simulink model "HLS_VMC_testing"  (R2025a)
settings: Solver=VariableStepAuto  StartTime=0.0  StopTime=0.0001  RelTol=1e-3
InitFcn:
  | fs = 500e6;
values from neighbouring files (symbols this model uses):
  N = length(X)    [outputPlots.m]
undefined symbols (not defined in the file or in its folder): A, es1, i, S, vsva2488, xcvr1602
libraries: hdlBasic x98, hlsBasic x64, aieUtilities x18, dspsrcs4 x15, dspxfrm3 x2, hdlDSPIP x2, hlsUtilities x1, vmcUtilities x1
(part 1 of 4)
settings Model: Creator=froregan  LastModifiedBy=froregan

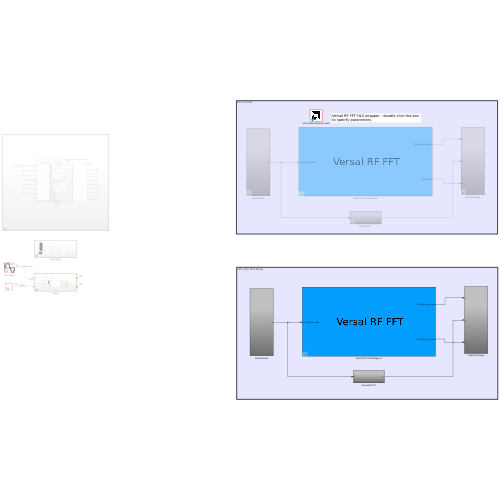
[thumbnail: Simulink's stored preview of the top-level diagram]
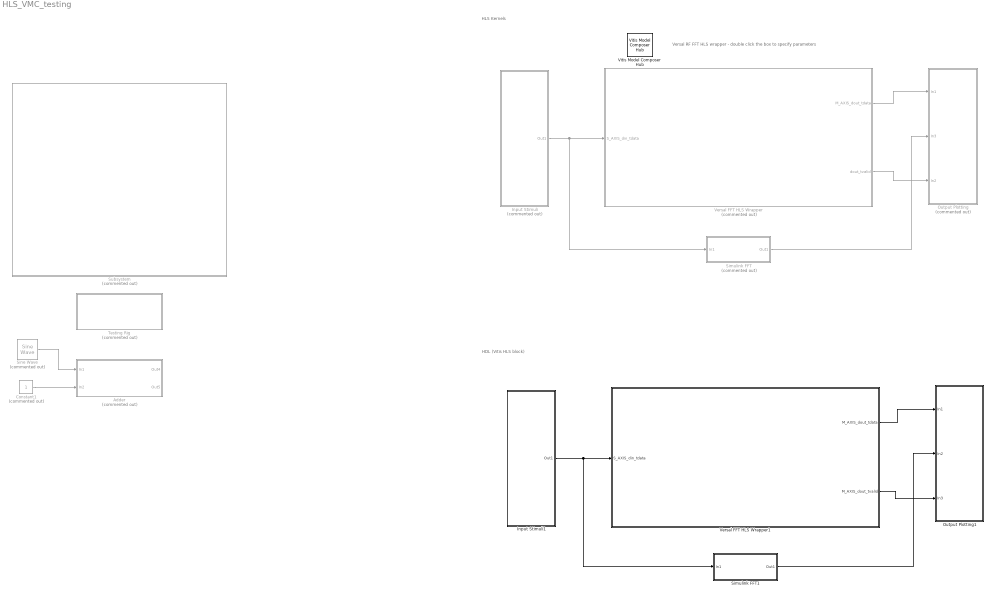
== system HLS_VMC_testing ==
  note: HDL (Vitis HLS block)
  note: HLS Kernels
  note: Versal RF FFT HLS wrapper - double click the box to specify parameters
  Adder : Subsystem  Commented=on
  Constant1 : Constant  Commented=on
  Input Stimuli : Subsystem  Commented=on
  Input Stimuli1 : Subsystem
  Output Plotting : Subsystem  Commented=on
  Output Plotting1 : Subsystem
  Simulink FFT : Subsystem  Commented=on
  Simulink FFT1 : Subsystem
  Sine Wave : dspsrcs4/Sine Wave  Commented=on  Amplitude=1  Frequency=100e6  Phase=0  SampleMode=Discrete  OutComplex=Real  CompMethod=Trigonometric fcn  TableSize=Speed  SampleTime=1/fs  SamplesPerFrame=1  ResetState=Restart at time zero  OutputFrames=off  dataType=double  wordLen=16  udDataType=sfix(16)  fracBitsMode=Best precision  numFracBits=15  OutDataTypeStr=double  LastOutDataTypeStr=double
  Subsystem : Subsystem  Commented=on
  Testing Rig : Subsystem  Commented=on
  Versal FFT HLS Wrapper : Subsystem  Commented=on  mask{tuser=1/1024, tuser_dir=IFFT, tuser_ps=10, FFT_SIZE=1024, sample_rate=SSR4, fft_max_point_size_temp=1024}
      mask prompts: tuser "TUSER Scaling"; tuser_dir "FFT Direction"; tuser_ps "TUSER Point Size"; FFT_SIZE "Period"; sample_rate "Super Sample Rate"; fft_max_point_size_temp "Maximum FFT Point Size"
      mask TypeOptions sample_rate: SSR2 | SSR4 | SSR8
      mask TypeOptions fft_max_point_size_temp: 16 | 32 | 64 | 128 | 256 | 512 | 1024 | 2048 | 4096
      mask DialogControl DescGroupVar Prompt: TUSER
      mask DialogControl Control4 Prompt: TUSER Scaling scales the output of the FFT
      mask DialogControl DescTextVar Prompt: TUSER Direction is either 1 for FFT or 0 for IFFT
      mask DialogControl Control3 Prompt: TUSER Point size is N where 2^N is the max FFT point size
      mask DialogControl ParameterGroupVar Prompt: TLAST
      mask DialogControl Control2 Prompt: Should be the same as the FFT size (in samples)
      mask DialogControl Container3 Prompt: Versal RF FFT
  Versal FFT HLS Wrapper1 : Subsystem  mask{tuser=1/1024, tuser_dir=FFT, tuser_ps=10, FFT_SIZE=1024, sample_rate=SSR4, fft_max_point_size_temp=1024}
      mask prompts: tuser "Scaling"; tuser_dir "FFT Direction"; tuser_ps "Point Size"; FFT_SIZE "Period"; sample_rate "Super Sample Rate"; fft_max_point_size_temp "Maximum FFT Point Size"
      mask TypeOptions sample_rate: SSR2 | SSR4 | SSR8
      mask TypeOptions fft_max_point_size_temp: 16 | 32 | 64 | 128 | 256 | 512 | 1024 | 2048 | 4096
      mask DialogControl DescGroupVar Prompt: TUSER
      mask DialogControl Control4 Prompt: TUSER Scaling scales the output of the FFT
      mask DialogControl DescTextVar Prompt: TUSER Direction is either 1 for FFT or 0 for IFFT
      mask DialogControl Control3 Prompt: TUSER Point size is N where 2^N is the max FFT point size
      mask DialogControl ParameterGroupVar Prompt: TLAST
      mask DialogControl Control2 Prompt: Should be the same as the FFT size (in samples)
      mask DialogControl Container3 Prompt: Versal RF FFT
  Vitis Model Composer Hub : vmcUtilities/Vitis Model Composer Hub  Tag=genX  CodeGeneration=off  SubsystemName=Versal FFT HLS Wrapper1  BlockHierPath=HLS_VMC_testing/Versal FFT HLS Wrapper1  CompilationType=HDLCompilation  SubsystemType=HDLNode  ExportTypeV2=IP Catalog  StartColumn=1  NumberOfColumns=1  TargetDirectory=./netlist  exportDesign=on  analyzeDesign=off  validateDesignOnHw=off  ExportType=AI Engines  IpVendor=xilinx.com  IpLibrary=hls  IpVersion=1.0  IpHWLanguage=Verilog  AieCompilerOptions={}  AieSimulatorOptions={}  CreateTestbench=off  TestbenchStackSize=10  RunRtlSim=off  RunCSim=off  RunAieSim=off  AieSimTimeout=50000  RunAieSimProfiling=off  LaunchVitisAnalyzer=off  PlotOutput=off  RunX86Sim=off  X86SimTimeout=10  GenHwImage=off  GenLibadfXo=on  GenHwValidationCode=off  PlatformType=Not Specified  HwSystemType=Baremetal  HwValidationTarget=hw  ProjDevice=xcvr1602-vsva2488-2HP-i-S-es1  ProjDevicePart=xcvr1602-vsva2488-2HP-i-S-es1  AIEType=AIE  SamplePeriod=-1  ClockFrequency=200  DataPathParallelism=1  xilinxfamily=versalairfes1  part=xcvr1602  speed=-2HP-i-S-es1  package=vsva2488  directory=./netlist/ip/Versal_FFT_HLS_Wrapper1/src  testbench=off  incr_netlist=off  synthesis_tool=Vivado  clock_wrapper=Clock Enables  dbl_ovrd=According to Block Masks  dcm_input_clock_period=10  sysclk_period=2  simulink_period=1/fs  eval_field=0  IPInfoJsonString="{\"DUTSubsystemName\":\"Versal FFT HLS Wrapper1\",\"HDLSubsystem\":{\"SubsystemName\":\"Versal_FFT_HLS_Wrapper1\",\"IPName\":\"Versal_FFT_HLS_Wrapper1\",\"IPLibrary\":\"VMC\",\"IPVendor\":\"User Company\",\"IPVersion\":\"1.0\",\"TargetDirectory\":\"./netlist\",\"SubsystemDir\":\"./netlist/ip/Versal_FFT_HLS_Wrapper1\",\"FreqHz\":\"500000000\"},\"SubsystemTag\":\"HDLNode\"}"  LogFileName=/proj/xirhdstaff1/froregan/icd7n/hegd_froregan_vmc_versalrf/DEV/hw/vmc_versalrf/HLS/netlist/model_composer.log  NThreads=4  IPConfigFile=/tmp/vmctmp-7794271613498057694/HLS_VMC_testing_ipconfig.json
  wires:
  Sine Wave/1 -> Adder/1(In1)
  Constant1/1 -> Adder/2(In2)
  Input Stimuli/1(Out1) -> Simulink FFT/1(In1), Versal FFT HLS Wrapper/1(S_AXIS_din_tdata)
  Versal FFT HLS Wrapper/1(M_AXIS_dout_tdata) -> Output Plotting/1(In1)
  Versal FFT HLS Wrapper/2(dout_tvalid) -> Output Plotting/3(In2)
  Simulink FFT/1(Out1) -> Output Plotting/2(In3)
  Simulink FFT1/1(Out1) -> Output Plotting1/2(In2)
  Input Stimuli1/1(Out1) -> Simulink FFT1/1(In1), Versal FFT HLS Wrapper1/1(S_AXIS_din_tdata)
  Versal FFT HLS Wrapper1/1(M_AXIS_dout_tdata) -> Output Plotting1/1(In1)
  Versal FFT HLS Wrapper1/2(M_AXIS_dout_tvalid) -> Output Plotting1/3(In3)

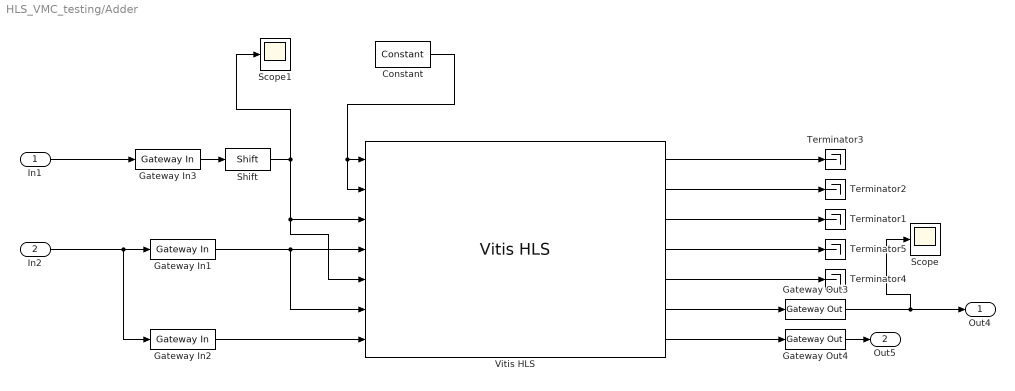
== system HLS_VMC_testing/Adder ==
  In1 : Inport
  In2 : Inport  Port=2
  Constant : hdlBasic/Constant  const=1.0  gui_display_data_type=Boolean  arith_type=Boolean  n_bits=16  bin_pt=14  preci_type=Single  exp_width=8  frac_width=24  explicit_period=off  period=1  XmcBlockStatus=1  maskContainerNames=tabcontainer1  block_type=constant  block_config=sysgen:Constant_config
  Gateway In1 : hdlBasic/Gateway In  gui_display_data_type=Boolean  arith_type=Boolean  n_bits=16  bin_pt=14  preci_type=Single  exp_width=8  frac_width=24  rows=1  columns=1  quantization="Round  (unbiased: +/- Inf)"  overflow=Saturate  period=1/fs  UseAsADC=off  ADCChannel='1'  interface=None  automatic_assignment=on  address_offset=hex2dec('00')  intf_name=''  intf_description=''  default_value=0  timing_constraint=None  locs_specified=off  LOCs={}  io_standard={}  inherit_from_input=off  hdl_port=on  XmcBlockStatus=1  maskContainerNames=group4  block_type=gatewayin  block_config=sysgen:gateway_in_config  block_width_w=590  block_height_w=620  block_width=640  block_height=850
  Gateway In2 : hdlBasic/Gateway In  gui_display_data_type=Boolean  arith_type=Boolean  n_bits=16  bin_pt=14  preci_type=Single  exp_width=8  frac_width=24  rows=1  columns=1  quantization="Round  (unbiased: +/- Inf)"  overflow=Saturate  period=1/fs  UseAsADC=off  ADCChannel='1'  interface=None  automatic_assignment=on  address_offset=hex2dec('00')  intf_name=''  intf_description=''  default_value=0  timing_constraint=None  locs_specified=off  LOCs={}  io_standard={}  inherit_from_input=off  hdl_port=on  XmcBlockStatus=1  maskContainerNames=group4  block_type=gatewayin  block_config=sysgen:gateway_in_config  block_width_w=590  block_height_w=620  block_width=640  block_height=850
  Gateway In3 : hdlBasic/Gateway In  gui_display_data_type=Fixed-point  arith_type=Signed (2's comp)  n_bits=32  bin_pt=31  preci_type=Single  exp_width=8  frac_width=24  rows=1  columns=1  quantization="Round  (unbiased: +/- Inf)"  overflow=Saturate  period=1/fs  UseAsADC=off  ADCChannel='1'  interface=None  automatic_assignment=on  address_offset=hex2dec('00')  intf_name=''  intf_description=''  default_value=0  timing_constraint=None  locs_specified=off  LOCs={}  io_standard={}  inherit_from_input=off  hdl_port=on  XmcBlockStatus=1  maskContainerNames=group4  block_type=gatewayin  block_config=sysgen:gateway_in_config  block_width_w=590  block_height_w=620  block_width=640  block_height=850
  Gateway Out3 : hdlBasic/Gateway Out  inherit_from_input=off  bool_to_boolean=off  hdl_port=on  rows=1  columns=1  UseAsDAC=off  DACChannel='1'  interface=None  automatic_assignment=on  address_offset=hex2dec('00')  intf_name=''  intf_description=''  timing_constraint=None  locs_specified=off  LOCs={}  io_standard={}  XmcBlockStatus=1  maskContainerNames=group4  block_type=gatewayout  block_config=sysgen:gateway_out_config  block_width_w=590  block_height_w=620  block_width=620  block_height=750
  Gateway Out4 : hdlBasic/Gateway Out  inherit_from_input=off  bool_to_boolean=off  hdl_port=on  rows=1  columns=1  UseAsDAC=off  DACChannel='1'  interface=None  automatic_assignment=on  address_offset=hex2dec('00')  intf_name=''  intf_description=''  timing_constraint=None  locs_specified=off  LOCs={}  io_standard={}  XmcBlockStatus=1  maskContainerNames=group4  block_type=gatewayout  block_config=sysgen:gateway_out_config  block_width_w=590  block_height_w=620  block_width=620  block_height=750
  Scope : Scope
      settings: ActiveDisplayYMinimum=-2.213061075E+9  ActiveDisplayYMaximum=2.213061075E+9  DataLoggingVariableName=ScopeData24
  Scope1 : Scope
      settings: ActiveDisplayYMinimum=-2.55297289625E+9  ActiveDisplayYMaximum=2.55297289625E+9  DataLoggingVariableName=ScopeData8
  Shift : hdlBasic/Shift  shift_dir=Left  shift_bits=31  en=off  latency=0  precision=User Defined  arith_type="Signed  (2's comp)"  n_bits=32  bin_pt=0  quantization=Truncate  overflow=Wrap  XmcBlockStatus=1  maskContainerNames=group2  block_type=shift  block_config=sysgen:Shift_config
  Terminator{1..5} (5 alike) : Terminator
  Vitis HLS : hdlBasic/Vitis HLS  anytable='/proj/xirhdstaff1/froregan/icd7n/hegd_froregan_vmc_versalrf/DEV/hw/vmc_versalrf/HLS/adder/adder/hls'  fast_sim=off  display_datatype=on  rate_propagation_method=Simulink system period  model_file_path=''  latency=1  block_type=vitis_hls
      settings: infoedit=This block allows including C,C++ and SystemC source files in System Generator for DSP designs.
  Out4 : Outport
  Out5 : Outport  Port=2
  wires:
  In1/1 -> Gateway In3/1
  In2/1 -> Gateway In2/1, Gateway In1/1
  Gateway In1/1 -> Vitis HLS/6, Vitis HLS/4
  Gateway In3/1 -> Shift/1
  Gateway In2/1 -> Vitis HLS/7
  Vitis HLS/6 -> Gateway Out3/1
  Gateway Out3/1 -> Scope/1, Out4/1
  Vitis HLS/7 -> Gateway Out4/1
  Gateway Out4/1 -> Out5/1
  Vitis HLS/2 -> Terminator2/1
  Vitis HLS/3 -> Terminator1/1
  Vitis HLS/1 -> Terminator3/1
  Vitis HLS/4 -> Terminator5/1
  Vitis HLS/5 -> Terminator4/1
  Shift/1 -> Vitis HLS/5, Vitis HLS/3, Scope1/1
  Constant/1 -> Vitis HLS/1, Vitis HLS/2

== system HLS_VMC_testing/Input Stimuli ==
  Chirp : dspsrcs4/Chirp  sweep=Quadratic  mode=Unidirectional  f0=100e3  f1=150e6  t1=1024/fs  Tsweep=1024/fs  phase=0  Ts=1/fs  spf=1  datatype=double  OutputFrames=off
  Chirp2 : dspsrcs4/Chirp  sweep=Quadratic  mode=Unidirectional  f0=100e3  f1=150e6  t1=1024/fs  Tsweep=1024/fs  phase=pi  Ts=1/fs  spf=1  datatype=double  OutputFrames=off
  Real-Imag to Complex : RealImagToComplex
  Sine Wave : dspsrcs4/Sine Wave  Commented=on  Amplitude=1  Frequency=100e3  Phase=0  SampleMode=Discrete  OutComplex=Complex  CompMethod=Trigonometric fcn  TableSize=Speed  SampleTime=1/fs  SamplesPerFrame=1  ResetState=Restart at time zero  OutputFrames=off  dataType=double  wordLen=16  udDataType=sfix(16)  fracBitsMode=Best precision  numFracBits=15  OutDataTypeStr=double  LastOutDataTypeStr=double
  Spectrum Analyzer : SpectrumAnalyzer  WindowPosition=[880.000000,470.000000,800.000000,500.000000,]  ScopeFrameLocation=window  WindowInvariantSamplesPerUpdate=on  Span=499999999.99999994  StartFrequency=-249999999.99999997  StopFrequency=249999999.99999997  YLimits=[-48.7308 24.4928]
  Out1 : Outport
  wires:
  Chirp2/1 -> Real-Imag to Complex/2
  Chirp/1 -> Real-Imag to Complex/1
  Real-Imag to Complex/1 -> Spectrum Analyzer/1, Out1/1

== system HLS_VMC_testing/Input Stimuli1 ==
  Chirp : dspsrcs4/Chirp  sweep=Quadratic  mode=Unidirectional  f0=100e3  f1=150e6  t1=1024/fs  Tsweep=1024/fs  phase=0  Ts=1/fs  spf=1  datatype=double  OutputFrames=off
  Chirp2 : dspsrcs4/Chirp  sweep=Quadratic  mode=Unidirectional  f0=100e3  f1=150e6  t1=1024/fs  Tsweep=1024/fs  phase=pi  Ts=1/fs  spf=1  datatype=double  OutputFrames=off
  Pre Processing : Subsystem
  Scope : Scope
      settings: ActiveDisplayYMinimum=-1.1949385808320478  ActiveDisplayYMaximum=1.2438820645368942  DataLoggingVariableName=ScopeData12
  Sine Wave : dspsrcs4/Sine Wave  Amplitude=1  Frequency=100e6  Phase=0  SampleMode=Discrete  OutComplex=Complex  CompMethod=Trigonometric fcn  TableSize=Speed  SampleTime=1/fs  SamplesPerFrame=1  ResetState=Restart at time zero  OutputFrames=off  dataType=double  wordLen=16  udDataType=sfix(16)  fracBitsMode=Best precision  numFracBits=15  OutDataTypeStr=double  LastOutDataTypeStr=double
  Spectrum Analyzer : SpectrumAnalyzer  WindowPosition=[880.000000,470.000000,800.000000,500.000000,]  ScopeFrameLocation=window  WindowInvariantSamplesPerUpdate=on  Span=999999999.9999999  StartFrequency=-499999999.99999994  StopFrequency=499999999.99999994  YLimits=[-44.7745 38.0195]
  Out1 : Outport
  wires:
  Pre Processing/1(HDL_FFT) -> Out1/1, Spectrum Analyzer/1, Scope/1
  Sine Wave/1 -> Pre Processing/1(In1)

== system HLS_VMC_testing/Output Plotting ==
  In1 : Inport
  In3 : Inport  Port=2
  In2 : Inport  Port=3
  Array Plot : ArrayPlot  WindowPosition=[6.000000,26.000000,1920.000000,1029.000000,]  ScopeFrameLocation=window  YLimits=[0.2195 0.2823]
  Scope : Scope
      settings: ActiveDisplayYMinimum=-0.032850187970989347  ActiveDisplayYMaximum=0.29565169173890421  DataLoggingVariableName=ScopeData7
  Scope1 : Scope
      settings: ActiveDisplayYMinimum=-0.33531683629605624  ActiveDisplayYMaximum=0.343925490006104  DataLoggingVariableName=ScopeData13
  Subsystem : Subsystem
  To File : ToFile  SaveFormat=Timeseries
  To Workspace : ToWorkspace  VariableName=fft  SaveFormat=Structure With Time  SampleTime=-1
  wires:
  Subsystem/1(Out1) -> Scope/1, Array Plot/1
  In2/1 -> Subsystem/Enable
  In1/1 -> To File/1, Scope1/1, To Workspace/1, Subsystem/1(In1)

== system HLS_VMC_testing/Output Plotting1 ==
  In1 : Inport
  In2 : Inport  Port=2
  In3 : Inport  Port=3
  Array Plot : ArrayPlot  WindowPosition=[1.000000,1.000000,2560.000000,1389.000000,]  ScopeFrameLocation=window  YLimits=[-10 10]
  Data Type Conversion : hlsBasic/Data Type Conversion  OutDataType=double  TypeExp=''  Signedness=Signed  WordLength=16  FractionalLength=0  RoundingMode=Truncation to minus infinity  OverflowMode=Wrap around
  Scope : Scope
      settings: ActiveDisplayYMinimum=-4.21288427541389E+36  ActiveDisplayYMaximum=3.7915958478725025E+37  DataLoggingVariableName=ScopeData7
  Scope1 : Scope
      settings: ActiveDisplayYMinimum=-5.8908108701306883E+37  ActiveDisplayYMaximum=5.1701277826062239E+37  DataLoggingVariableName=ScopeData18
  Subsystem : Subsystem
  To Workspace : ToWorkspace  VariableName=fft  SaveFormat=Timeseries  SampleTime=-1
  To Workspace1 : ToWorkspace  VariableName=simulink  SaveFormat=Timeseries  SampleTime=-1
  wires:
  In1/1 -> Data Type Conversion/1
  Subsystem/1(Out1) -> Scope/1, Array Plot/1, To Workspace/1
  Data Type Conversion/1 -> Scope1/1, Subsystem/1(In1)
  In2/1 -> To Workspace1/1

== system HLS_VMC_testing/Simulink FFT ==
  In1 : Inport
  Abs : Abs  SaturateOnIntegerOverflow=off
  Buffer : Buffer  N=1024  OutputFrames=off
  FFT : dspxfrm3/FFT  FFTImplementation=Auto  CompMethod=Table lookup  TableOpt=NEW  TableOptActive=Speed  BitRevOrder=off  Normalize=off  InheritFFTLength=on  FFTLength=64  WrapInput=on  roundingMode=Ceiling  overflowMode=off  firstCoeffDataTypeStr=Inherit: Same word length as input  firstCoeffLastDataTypeStr=Inherit: Same word length as input  outputMin=[]  outputMax=[]
  Out1 : Outport
  wires:
  Buffer/1 -> FFT/1
  FFT/1 -> Abs/1
  In1/1 -> Buffer/1
  Abs/1 -> Out1/1

== system HLS_VMC_testing/Simulink FFT1 ==
  In1 : Inport
  Abs : Abs  SaturateOnIntegerOverflow=off
  Buffer : Buffer  N=1024  OutputFrames=off
  FFT : dspxfrm3/FFT  FFTImplementation=Auto  CompMethod=Table lookup  TableOpt=NEW  TableOptActive=Speed  BitRevOrder=off  Normalize=off  InheritFFTLength=on  FFTLength=64  WrapInput=on  roundingMode=Ceiling  overflowMode=off  firstCoeffDataTypeStr=Inherit: Same word length as input  firstCoeffLastDataTypeStr=Inherit: Same word length as input  outputMin=[]  outputMax=[]
  Out1 : Outport
  wires:
  Buffer/1 -> FFT/1
  FFT/1 -> Abs/1
  In1/1 -> Buffer/1
  Abs/1 -> Out1/1

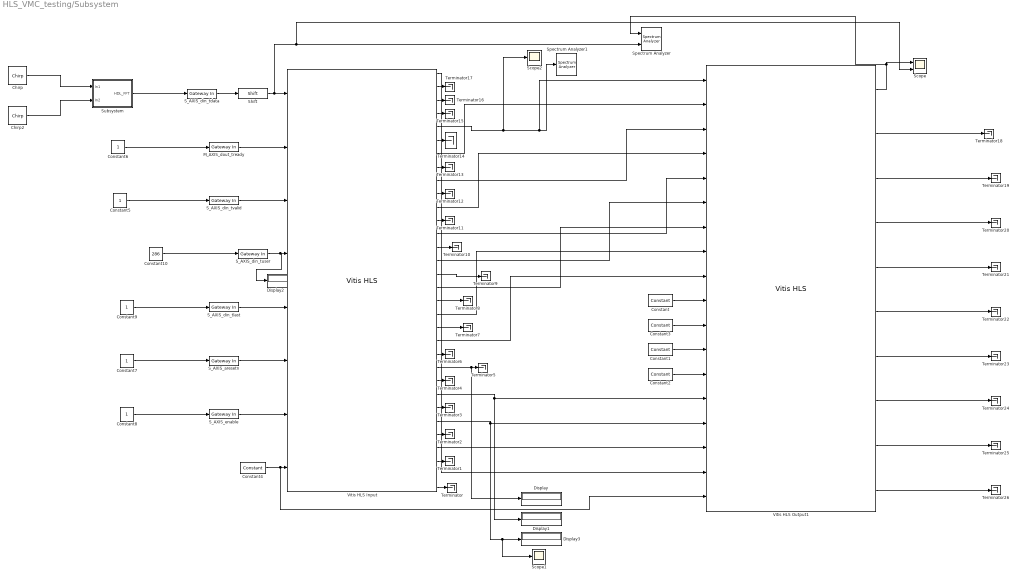
== system HLS_VMC_testing/Subsystem ==
  Chirp : dspsrcs4/Chirp  sweep=Quadratic  mode=Unidirectional  f0=100e3  f1=150e6  t1=1024/fs  Tsweep=1024/fs  phase=0  Ts=1/fs  spf=1  datatype=double  OutputFrames=off
  Chirp2 : dspsrcs4/Chirp  sweep=Quadratic  mode=Unidirectional  f0=100e3  f1=150e6  t1=1024/fs  Tsweep=1024/fs  phase=pi  Ts=1/fs  spf=1  datatype=double  OutputFrames=off
  Constant{,1..3} (4 alike) : hdlBasic/Constant  const=1.0  gui_display_data_type=Fixed-point  arith_type=Unsigned  n_bits=12  bin_pt=0  preci_type=Single  exp_width=8  frac_width=24  explicit_period=off  period=1  XmcBlockStatus=1  maskContainerNames=tabcontainer1  block_type=constant  block_config=sysgen:Constant_config
  Constant10 : Constant  Value=286
  Constant4 : hdlBasic/Constant  const=0  gui_display_data_type=Boolean  arith_type=Boolean  n_bits=16  bin_pt=14  preci_type=Single  exp_width=8  frac_width=24  explicit_period=off  period=1  XmcBlockStatus=1  maskContainerNames=tabcontainer1  block_type=constant  block_config=sysgen:Constant_config
  Constant{5..9} (5 alike) : Constant
  Display{,1..3} (4 alike) : Display
  M_AXIS_dout_tready : hdlBasic/Gateway In  gui_display_data_type=Boolean  arith_type=Boolean  n_bits=16  bin_pt=14  preci_type=Single  exp_width=8  frac_width=24  rows=1  columns=1  quantization="Round  (unbiased: +/- Inf)"  overflow=Saturate  period=1/fs  UseAsADC=off  ADCChannel='1'  interface=None  automatic_assignment=on  address_offset=hex2dec('00')  intf_name=''  intf_description=''  default_value=0  timing_constraint=None  locs_specified=off  LOCs={}  io_standard={}  inherit_from_input=off  hdl_port=on  XmcBlockStatus=1  maskContainerNames=group4  block_type=gatewayin  block_config=sysgen:gateway_in_config  block_width_w=590  block_height_w=620  block_width=640  block_height=850
  S_AXIS_aresetn : hdlBasic/Gateway In  gui_display_data_type=Boolean  arith_type=Boolean  n_bits=16  bin_pt=14  preci_type=Single  exp_width=8  frac_width=24  rows=1  columns=1  quantization="Round  (unbiased: +/- Inf)"  overflow=Saturate  period=1/fs  UseAsADC=off  ADCChannel='1'  interface=None  automatic_assignment=on  address_offset=hex2dec('00')  intf_name=''  intf_description=''  default_value=0  timing_constraint=None  locs_specified=off  LOCs={}  io_standard={}  inherit_from_input=off  hdl_port=on  XmcBlockStatus=1  maskContainerNames=group4  block_type=gatewayin  block_config=sysgen:gateway_in_config  block_width_w=590  block_height_w=620  block_width=640  block_height=850
  S_AXIS_din_tdata : hdlBasic/Gateway In  gui_display_data_type=Fixed-point  arith_type=Signed (2's comp)  n_bits=128  bin_pt=127  preci_type=Single  exp_width=8  frac_width=24  rows=1  columns=1  quantization="Round  (unbiased: +/- Inf)"  overflow=Saturate  period=1/fs  UseAsADC=off  ADCChannel='1'  interface=None  automatic_assignment=on  address_offset=hex2dec('00')  intf_name=''  intf_description=''  default_value=0  timing_constraint=None  locs_specified=off  LOCs={}  io_standard={}  inherit_from_input=off  hdl_port=on  XmcBlockStatus=1  maskContainerNames=group4  block_type=gatewayin  block_config=sysgen:gateway_in_config  block_width_w=590  block_height_w=620  block_width=640  block_height=850
  S_AXIS_din_tlast : hdlBasic/Gateway In  gui_display_data_type=Boolean  arith_type=Boolean  n_bits=16  bin_pt=14  preci_type=Single  exp_width=8  frac_width=24  rows=1  columns=1  quantization="Round  (unbiased: +/- Inf)"  overflow=Saturate  period=1/fs  UseAsADC=off  ADCChannel='1'  interface=None  automatic_assignment=on  address_offset=hex2dec('00')  intf_name=''  intf_description=''  default_value=0  timing_constraint=None  locs_specified=off  LOCs={}  io_standard={}  inherit_from_input=off  hdl_port=on  XmcBlockStatus=1  maskContainerNames=group4  block_type=gatewayin  block_config=sysgen:gateway_in_config  block_width_w=590  block_height_w=620  block_width=640  block_height=850
  S_AXIS_din_tuser : hdlBasic/Gateway In  gui_display_data_type=Fixed-point  arith_type=Unsigned  n_bits=18  bin_pt=0  preci_type=Single  exp_width=8  frac_width=24  rows=1  columns=1  quantization="Round  (unbiased: +/- Inf)"  overflow=Saturate  period=1/fs  UseAsADC=off  ADCChannel='1'  interface=None  automatic_assignment=on  address_offset=hex2dec('00')  intf_name=''  intf_description=''  default_value=0  timing_constraint=None  locs_specified=off  LOCs={}  io_standard={}  inherit_from_input=off  hdl_port=on  XmcBlockStatus=1  maskContainerNames=group4  block_type=gatewayin  block_config=sysgen:gateway_in_config  block_width_w=590  block_height_w=620  block_width=640  block_height=850
  S_AXIS_din_tvalid : hdlBasic/Gateway In  gui_display_data_type=Boolean  arith_type=Boolean  n_bits=16  bin_pt=14  preci_type=Single  exp_width=8  frac_width=24  rows=1  columns=1  quantization="Round  (unbiased: +/- Inf)"  overflow=Saturate  period=1/fs  UseAsADC=off  ADCChannel='1'  interface=None  automatic_assignment=on  address_offset=hex2dec('00')  intf_name=''  intf_description=''  default_value=0  timing_constraint=None  locs_specified=off  LOCs={}  io_standard={}  inherit_from_input=off  hdl_port=on  XmcBlockStatus=1  maskContainerNames=group4  block_type=gatewayin  block_config=sysgen:gateway_in_config  block_width_w=590  block_height_w=620  block_width=640  block_height=850
  S_AXIS_enable : hdlBasic/Gateway In  gui_display_data_type=Boolean  arith_type=Boolean  n_bits=16  bin_pt=14  preci_type=Single  exp_width=8  frac_width=24  rows=1  columns=1  quantization="Round  (unbiased: +/- Inf)"  overflow=Saturate  period=1/fs  UseAsADC=off  ADCChannel='1'  interface=None  automatic_assignment=on  address_offset=hex2dec('00')  intf_name=''  intf_description=''  default_value=0  timing_constraint=None  locs_specified=off  LOCs={}  io_standard={}  inherit_from_input=off  hdl_port=on  XmcBlockStatus=1  maskContainerNames=group4  block_type=gatewayin  block_config=sysgen:gateway_in_config  block_width_w=590  block_height_w=620  block_width=640  block_height=850
  Scope : Scope  NumInputPorts=2
      settings: ActiveDisplayYMinimum=-2.1267647932297024E+38  ActiveDisplayYMaximum=2.1267647932529583E+38  DataLoggingVariableName=ScopeData15
  Scope1 : Scope
      settings: ActiveDisplayYMinimum=-1  ActiveDisplayYMaximum=1  DataLoggingVariableName=ScopeData16
  Scope2 : Scope
      settings: ActiveDisplayYMinimum=-1  ActiveDisplayYMaximum=1  DataLoggingVariableName=ScopeData17
  Shift : hdlBasic/Shift  shift_dir=Left  shift_bits=127  en=off  latency=0  precision=User Defined  arith_type="Signed  (2's comp)"  n_bits=128  bin_pt=0  quantization="Round  (unbiased: +/- Inf)"  overflow=Saturate  XmcBlockStatus=1  maskContainerNames=group2  block_type=shift  block_config=sysgen:Shift_config
  Spectrum Analyzer : SpectrumAnalyzer  NumInputPorts=2  WindowPosition=[560.000000,290.000000,800.000000,500.000000,]  ScopeFrameLocation=window  WindowInvariantSamplesPerUpdate=on  Span=499999999.99999994  StartFrequency=-249999999.99999997  StopFrequency=249999999.99999997  YLimits=[723.8982 779.0019]
  Spectrum Analyzer1 : SpectrumAnalyzer  WindowPosition=[288.000000,6.000000,800.000000,500.000000,]  ScopeFrameLocation=window  WindowInvariantSamplesPerUpdate=on  YLimits=[-3603.4449 -2802.6794]
  Subsystem : Subsystem
  Terminator{,1..26} (27 alike) : Terminator
  Vitis HLS Input : hdlBasic/Vitis HLS  anytable='./new_wrapperIN/wrapperin/wrapperin/hls'  fast_sim=off  display_datatype=on  rate_propagation_method=Simulink system period  model_file_path=''  latency=1  block_type=vitis_hls
      settings: infoedit=This block allows including C,C++ and SystemC source files in System Generator for DSP designs.
  Vitis HLS Output1 : hdlBasic/Vitis HLS  anytable='./wrapper_out/wrapper_out/wrapper_out/hls'  fast_sim=off  display_datatype=on  rate_propagation_method=Simulink system period  model_file_path=''  latency=1  block_type=vitis_hls
      settings: infoedit=This block allows including C,C++ and SystemC source files in System Generator for DSP designs.
  wires:
  Vitis HLS Input/12 -> Terminator11/1
  Vitis HLS Output1/1 -> Spectrum Analyzer/1, Scope/1
  Vitis HLS Input/27 -> Scope1/1, Display3/1, Vitis HLS Output1/15
  Vitis HLS Input/1 -> Vitis HLS Output1/17
  Vitis HLS Input/20 -> Terminator7/1
  Vitis HLS Input/16 -> Terminator9/1
  Vitis HLS Input/32 -> Terminator/1
  Vitis HLS Input/30 -> Terminator1/1
  Vitis HLS Input/29 -> Vitis HLS Output1/16
  Vitis HLS Input/8 -> Terminator13/1
  Vitis HLS Input/28 -> Terminator2/1
  Vitis HLS Input/18 -> Terminator8/1
  Vitis HLS Input/4 -> Terminator15/1
  Vitis HLS Input/14 -> Terminator10/1
  Vitis HLS Input/26 -> Terminator3/1
  Vitis HLS Input/21 -> Vitis HLS Output1/9
  Vitis HLS Input/3 -> Terminator16/1
  Vitis HLS Input/22 -> Terminator6/1
  Vitis HLS Input/25 -> Display1/1, Vitis HLS Output1/14
  Vitis HLS Input/24 -> Terminator4/1
  Vitis HLS Input/23 -> Display/1, Terminator5/1
  Vitis HLS Input/10 -> Terminator12/1
  Vitis HLS Input/2 -> Terminator17/1
  Vitis HLS Input/6 -> Terminator14/1
  Vitis HLS Input/5 -> Scope2/1, Vitis HLS Output1/1, Spectrum Analyzer1/1
  Subsystem/1(HDL_FFT) -> S_AXIS_din_tdata/1
  Constant4/1 -> Vitis HLS Output1/18, Vitis HLS Input/8
  S_AXIS_din_tuser/1 -> Display2/1, Vitis HLS Input/4
  S_AXIS_enable/1 -> Vitis HLS Input/7
  S_AXIS_aresetn/1 -> Vitis HLS Input/6
  Constant6/1 -> M_AXIS_dout_tready/1
  S_AXIS_din_tvalid/1 -> Vitis HLS Input/3
  M_AXIS_dout_tready/1 -> Vitis HLS Input/2
  Constant5/1 -> S_AXIS_din_tvalid/1
  Constant8/1 -> S_AXIS_enable/1
  S_AXIS_din_tdata/1 -> Shift/1
  S_AXIS_din_tlast/1 -> Vitis HLS Input/5
  Constant9/1 -> S_AXIS_din_tlast/1
  Constant10/1 -> S_AXIS_din_tuser/1
  Constant7/1 -> S_AXIS_aresetn/1
  Constant/1 -> Vitis HLS Output1/10
  Constant1/1 -> Vitis HLS Output1/12
  Constant2/1 -> Vitis HLS Output1/13
  Constant3/1 -> Vitis HLS Output1/11
  Vitis HLS Output1/2 -> Terminator18/1
  Vitis HLS Output1/3 -> Terminator19/1
  Vitis HLS Output1/4 -> Terminator20/1
  Vitis HLS Output1/5 -> Terminator21/1
  Vitis HLS Output1/6 -> Terminator22/1
  Vitis HLS Output1/7 -> Terminator23/1
  Vitis HLS Output1/8 -> Terminator24/1
  Vitis HLS Output1/9 -> Terminator25/1
  Vitis HLS Output1/10 -> Terminator26/1
  Chirp2/1 -> Subsystem/2(In2)
  Chirp/1 -> Subsystem/1(In1)
  Vitis HLS Input/7 -> Vitis HLS Output1/2
  Vitis HLS Input/9 -> Vitis HLS Output1/3
  Vitis HLS Input/11 -> Vitis HLS Output1/4
  Vitis HLS Input/13 -> Vitis HLS Output1/5
  Vitis HLS Input/15 -> Vitis HLS Output1/6
  Vitis HLS Input/17 -> Vitis HLS Output1/7
  Vitis HLS Input/19 -> Vitis HLS Output1/8
  Shift/1 -> Vitis HLS Input/1, Scope/2, Spectrum Analyzer/2
